simulink model "hw4_q3"  (R2022b)
settings: Solver=VariableStepAuto  StartTime=0.0  StopTime=10.0  RelTol=1e-3
settings Model: Creator=shivavafadar  LastModifiedBy=shivavafadar

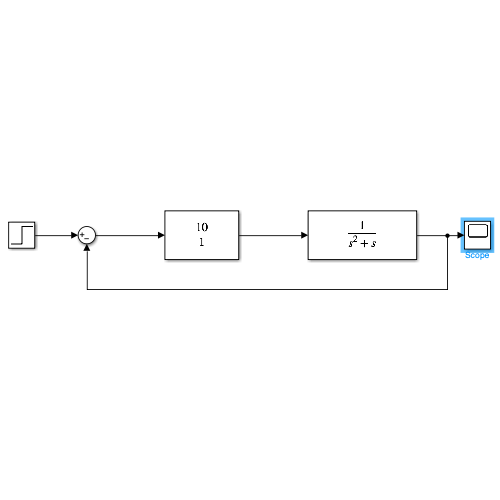
[thumbnail: Simulink's stored preview of the top-level diagram]
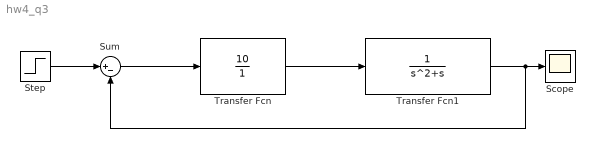
== system hw4_q3 ==
  Scope : Scope
  Step : Step  SampleTime=0
  Sum : Sum  Inputs=|+-
  Transfer Fcn : TransferFcn  Numerator=[10]  Denominator=[1]
  Transfer Fcn1 : TransferFcn  Denominator=[1 1 0]
  wires:
  Transfer Fcn/1 -> Transfer Fcn1/1
  Step/1 -> Sum/1
  Transfer Fcn1/1 -> Scope/1, Sum/2
  Sum/1 -> Transfer Fcn/1
